simulink model "W1Q4"  (R2020a)
settings: Solver=VariableStepAuto  StartTime=0.0  StopTime=10.0  RelTol=1e-3
settings Model: Creator=Vinayak  LastModifiedBy=Vinayak

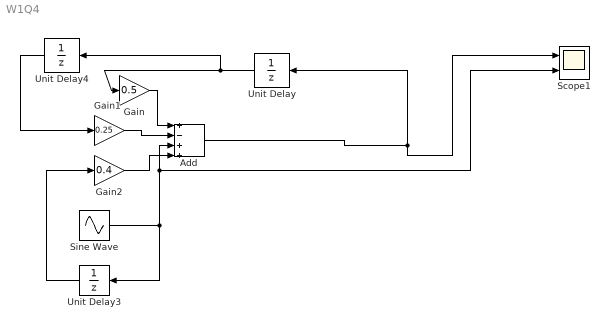
== system W1Q4 ==
  Add : Sum  Inputs=+-++
  Gain : Gain  Gain=0.5
  Gain1 : Gain  Gain=0.25
  Gain2 : Gain  Gain=0.4
  Scope1 : Scope  NumInputPorts=2
  Sine Wave : Sin  SampleTime=0
  Unit Delay : UnitDelay  SampleTime=-1  HasFrameUpgradeWarning=on
  Unit Delay3 : UnitDelay  SampleTime=-1  HasFrameUpgradeWarning=on
  Unit Delay4 : UnitDelay  SampleTime=-1  HasFrameUpgradeWarning=on
  wires:
  Add/1 -> Unit Delay/1, Scope1/1
  Unit Delay/1 -> Unit Delay4/1, Gain/1
  Gain/1 -> Add/1
  Gain2/1 -> Add/4
  Unit Delay3/1 -> Gain2/1
  Gain1/1 -> Add/2
  Unit Delay4/1 -> Gain1/1
  Sine Wave/1 -> Scope1/2, Add/3, Unit Delay3/1
